simulink model "example01"  (R2022a)
settings: Solver=VariableStepAuto  StartTime=0.0  StopTime=10.0  RelTol=1e-3
settings Model: Creator=cunis  LastModifiedBy=cunis

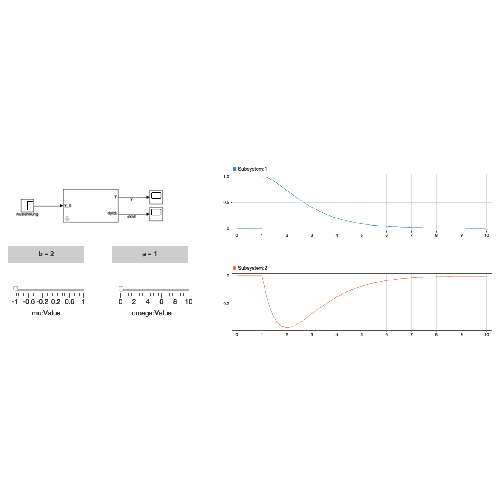
[thumbnail: Simulink's stored preview of the top-level diagram]
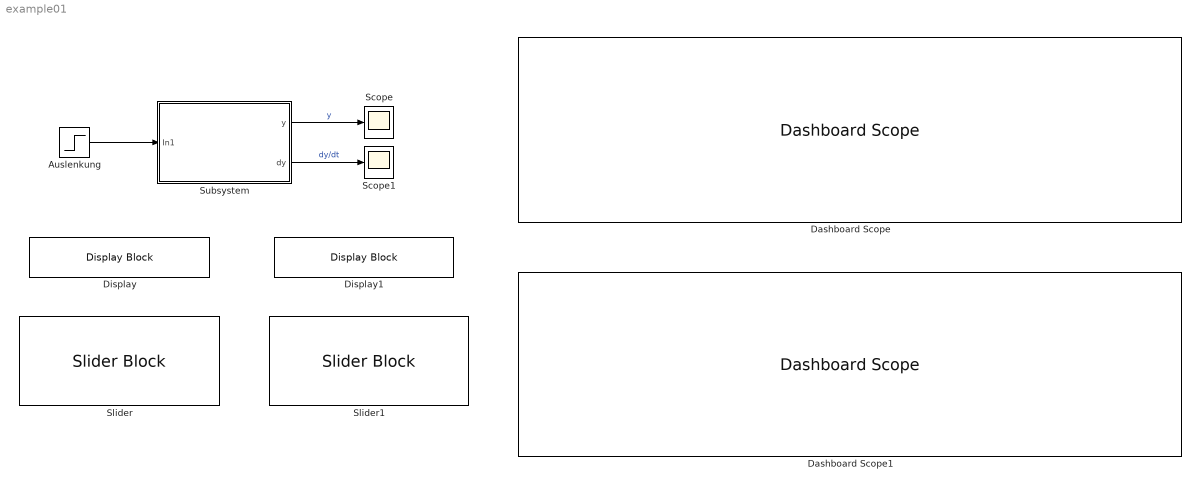
== system example01 ==
  Auslenkung : Step  SampleTime=0
  Dashboard Scope : DashboardScope
  Dashboard Scope1 : DashboardScope
  Display : DisplayBlock  LabelPosition=Hide  Format=Custom  Transparency=1  FormatString=b = %d
  Display1 : DisplayBlock  LabelPosition=Hide  Format=Custom  Transparency=1  FormatString=a = %d
  Scope : Scope
  Scope1 : Scope
  Slider : SliderBlock  LabelPosition=Bottom  ScaleMin=-1  ScaleMax=1
  Slider1 : SliderBlock  LabelPosition=Bottom  ScaleMax=10
  Subsystem : Subsystem
      mask Display:
      | port_label('input', 1, 'y_0');
      | port_label('output', 1, 'y');
      | port_label('output', 2, 'dy/dt');
  wires:
  Auslenkung/1 -> Subsystem/1(In1)
  Subsystem/1(y) -> Scope/1  "y"
  Subsystem/2(dy) -> Scope1/1  "dy/dt"

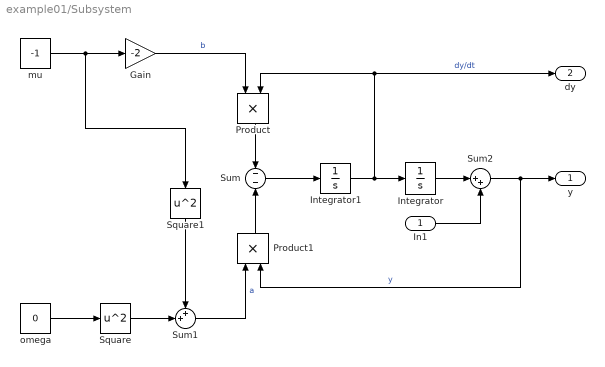
== system example01/Subsystem ==
  In1 : Inport
  Gain : Gain  Gain=-2
  Integrator : Integrator
  Integrator1 : Integrator
  Product : Product
  Product1 : Product
  Square : Math  Operator=square
  Square1 : Math  Operator=square
  Sum : Sum  Inputs=-|-
  Sum1 : Sum  Inputs=++|
  Sum2 : Sum  Inputs=|++
  mu : Constant  Value=-1
  omega : Constant  Value=0
  y : Outport
  dy : Outport  Port=2
  wires:
  In1/1 -> Sum2/2
  Sum2/1 -> Product1/2, y/1  "y"
  Integrator1/1 -> Product/2, dy/1, Integrator/1  "dy/dt"
  Sum/1 -> Integrator1/1
  Product/1 -> Sum/1
  Product1/1 -> Sum/2
  Gain/1 -> Product/1  "b"
  mu/1 -> Square1/1, Gain/1
  Sum1/1 -> Product1/1  "a"
  omega/1 -> Square/1
  Square1/1 -> Sum1/1
  Integrator/1 -> Sum2/1
  Square/1 -> Sum1/2
